simulink model "PENDULO_DOBLE"  (R2023b)
settings: Solver=VariableStepAuto  StartTime=0.0  StopTime=10.0  RelTol=1e-3
undefined symbols (not defined in the file): C, G
settings Model: Creator=Envy  LastModifiedBy=Envy

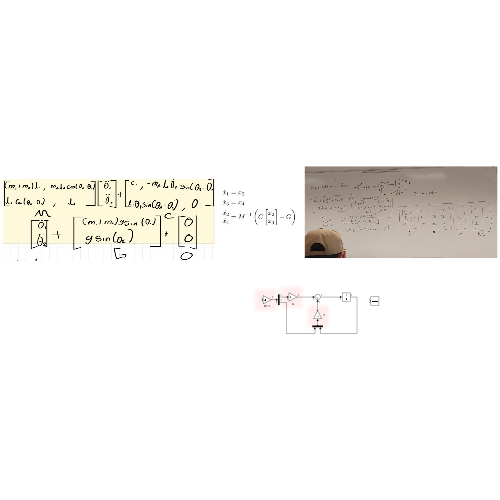
[thumbnail: Simulink's stored preview of the top-level diagram]
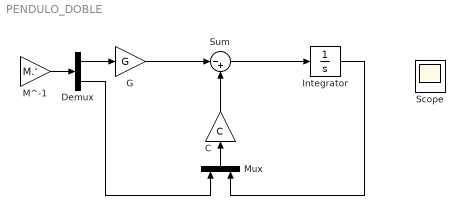
== system PENDULO_DOBLE ==
  C : Gain  Gain=C
  Demux : Demux  Outputs=2
  G : Gain  Gain=G
  Integrator : Integrator
  M^-1 : Gain  Gain=M.'
  Mux : Mux  Inputs=2
  Scope : Scope
  Sum : Sum  Inputs=|-+
  wires:
  Sum/1 -> Integrator/1
  G/1 -> Sum/1
  M^-1/1 -> Demux/1
  Demux/1 -> G/1
  C/1 -> Sum/2
  Mux/1 -> C/1
  Integrator/1 -> Mux/2
  Demux/2 -> Mux/1
